simulink model "shipdynamics"  (R2016b)
settings: Solver=ode45  StartTime=0.0  StopTime=50  RelTol=1e-3  EnableMultiTasking=on
settings Model: Creator=highamj  LastModifiedBy=chira
settings DataIOCC: LimitDataPoints=on  SaveFormat=Array
settings OptimizationCC: LifeSpan=inf
settings DebuggingCC: SolverPrmCheckMsg=warning  SFUnexpectedBacktrackingDiag=warning  SFNoUnconditionalDefaultTransitionDiag=warning  SFExecutionAtInitializationDiag=none
settings HardwareCC: ProdBitPerPointer=32  ProdBitPerSizeT=32  ProdBitPerPtrDiffT=32  ProdLargestAtomicFloat=None  ProdIntDivRoundTo=Undefined  ProdEndianess=Unspecified  ProdWordSize=32  ProdHWDeviceType=32-bit Generic
settings ModelReferenceCC: PropagateSignalLabelsOutOfModel=off
settings GRTTargetCC: TargetLangStandard=C89/C90 (ANSI)  GeneratePreprocessorConditionals=Disable all
settings ConfigComp: CovMetricSettings=dw  CovHtmlReporting=on  CovSaveCumulativeToWorkspaceVar=on  CovSaveSingleToWorkspaceVar=on  CovExternalEMLEnable=off  CovSFcnEnable=off

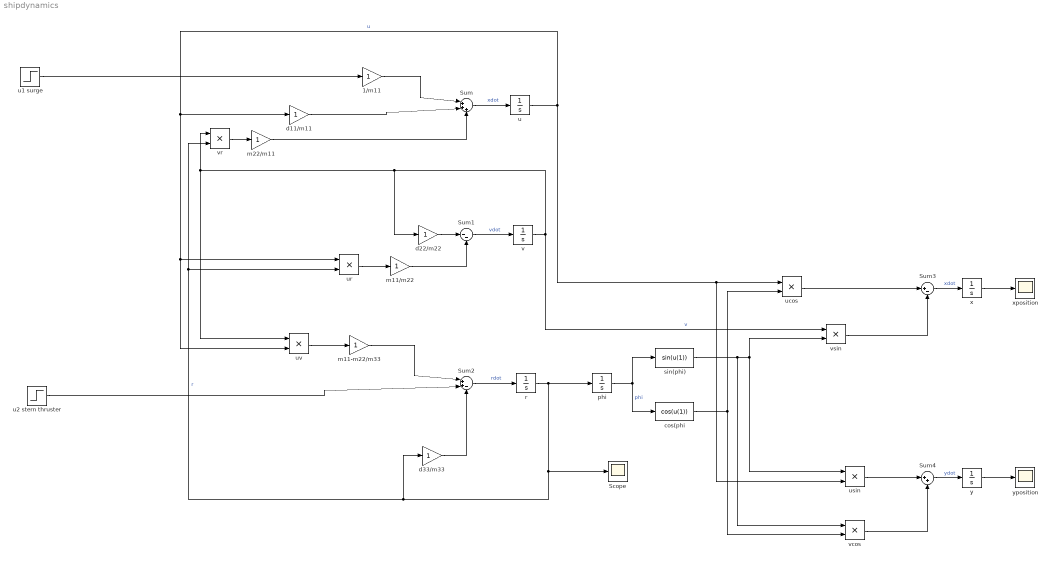
== system shipdynamics ==
  1/m11 : Gain
  Scope : Scope
  Sum : Sum  Inputs=|+++
  Sum1 : Sum  Inputs=|--
  Sum2 : Sum  Inputs=|++-
  Sum3 : Sum  Inputs=|+-
  Sum4 : Sum  Inputs=|++
  cos(phi : Fcn  Expr=cos(u(1))
  d11/m11 : Gain
  d22/m22 : Gain
  d33/m33 : Gain
  m11-m22/m33 : Gain
  m11/m22 : Gain
  m22/m11 : Gain
  phi : Integrator
  r : Integrator
  sin(phi) : Fcn  Expr=sin(u(1))
  u : Integrator
  u1 surge : Step  After=0  SampleTime=0
  u2 stern thruster : Step  Time=2  SampleTime=0
  ucos : Product
  ur : Product
  usin : Product
  uv : Product
  v : Integrator
  vcos : Product
  vr : Product
  vsin : Product
  x : Integrator
  xposition : Scope
  y : Integrator
  yposition : Scope
  wires:
  vr/1 -> m22/m11/1
  v/1 -> vsin/1, d22/m22/1, uv/1, vr/1  "v"
  r/1 -> phi/1, Scope/1, d33/m33/1, vr/2, ur/2  "r"
  Sum/1 -> u/1  "xdot"
  Sum1/1 -> v/1  "vdot"
  Sum2/1 -> r/1  "rdot"
  m22/m11/1 -> Sum/3
  u/1 -> uv/2, ur/1, d11/m11/1, usin/2, ucos/1  "u"
  d11/m11/1 -> Sum/2
  1/m11/1 -> Sum/1
  ur/1 -> m11/m22/1
  m11/m22/1 -> Sum1/2
  d22/m22/1 -> Sum1/1
  d33/m33/1 -> Sum2/3
  m11-m22/m33/1 -> Sum2/1
  uv/1 -> m11-m22/m33/1
  u1 surge/1 -> 1/m11/1
  u2 stern thruster/1 -> Sum2/2
  phi/1 -> sin(phi)/1, cos(phi/1  "phi"
  Sum4/1 -> y/1  "ydot"
  Sum3/1 -> x/1  "xdot"
  sin(phi)/1 -> vcos/1, vsin/2, usin/1
  cos(phi/1 -> vcos/2, ucos/2
  ucos/1 -> Sum3/1
  vsin/1 -> Sum3/2
  usin/1 -> Sum4/1
  vcos/1 -> Sum4/2
  x/1 -> xposition/1
  y/1 -> yposition/1
